simulink model "Task3_Gain"  (R2024b)
settings: Solver=VariableStepAuto  StartTime=0.0  StopTime=10.0  RelTol=1e-3
settings Model: Creator=Ahmad  LastModifiedBy=Ahmad

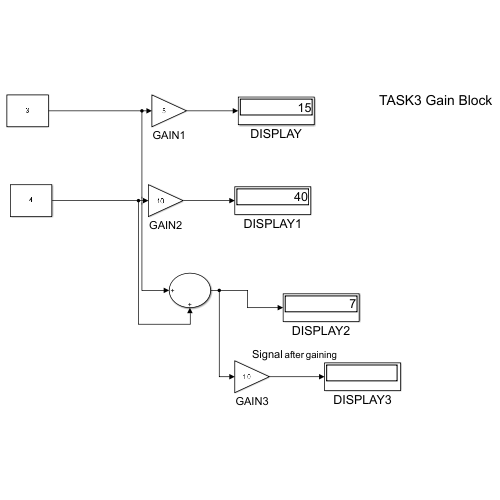
[thumbnail: Simulink's stored preview of the top-level diagram]
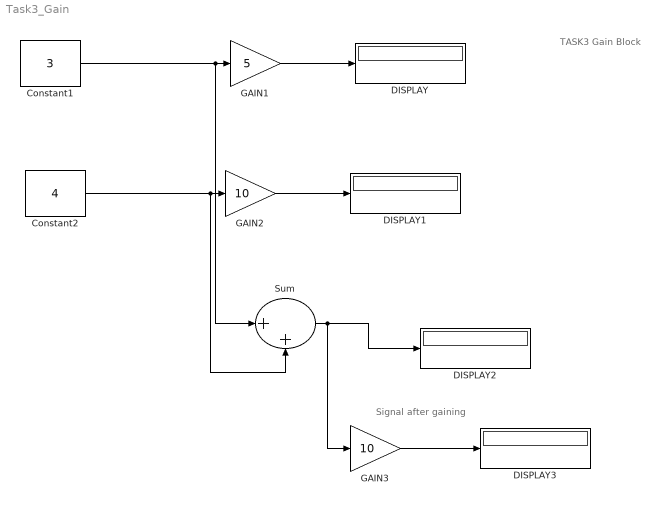
== system Task3_Gain ==
  note: TASK3 Gain Block
  note: Signal after gaining
  Constant1 : Constant  Value=3
  Constant2 : Constant  Value=4
  DISPLAY{,1..3} (4 alike) : Display
  GAIN1 : Gain  Gain=5
  GAIN2 : Gain  Gain=10
  GAIN3 : Gain  Gain=10
  Sum : Sum  Inputs=|++
  wires:
  Constant1/1 -> Sum/1, GAIN1/1
  GAIN1/1 -> DISPLAY/1
  Constant2/1 -> Sum/2, GAIN2/1
  GAIN2/1 -> DISPLAY1/1
  Sum/1 -> GAIN3/1, DISPLAY2/1
  GAIN3/1 -> DISPLAY3/1
